simulink model "KalmanFilterIMU"  (R2020a)
settings: Solver=FixedStepDiscrete  StartTime=0.0  StopTime=Inf  RelTol=1e-3
settings Model: SimulationMode=external  SILPILModeSetting=veronly  ExtModeTrigDuration=2  Creator=vishwasgautam  LastModifiedBy=vishwasgautam
settings OptimizationCC: EnhancedBackFolding=on  PassReuseOutputArgsAs=Individual arguments  ZeroExternalMemoryAtStartup=off  ZeroInternalMemoryAtStartup=off  MaxStackSize=64  OptimizeBlockOrder=speed  DifferentSizesBufferReuse=on  OptimizationCustomize=off  EfficientTunableParamExpr=on
settings DebuggingCC: ParameterTunabilityLossMsg=error
settings HardwareCC: ProdBitPerInt=16  ProdBitPerPointer=16  ProdBitPerSizeT=16  ProdBitPerPtrDiffT=16  ProdLargestAtomicFloat=None  ProdWordSize=8  ProdHWDeviceType=Atmel->AVR  UseEmbeddedCoderFeatures=off  UseSimulinkCoderFeatures=off
settings SFSimCC: MATLABDynamicMemAlloc=off
settings RTWCC: SystemTargetFile=ert.tlc  HardwareBoard=Arduino Uno  TLCOptions=-aInlineSetEventsForThisBaseRateFcn=TLC_FALSE -aSuppressMultiTaskScheduler=TLC_FALSE -aRateBasedStepFcn=1  TemplateMakefile=ert_default_tmf  Toolchain=Arduino AVR
settings CodeAppCC: ForceParamTrailComments=on  IgnoreCustomStorageClasses=off  OperatorAnnotations=on  SimulinkDataObjDesc=on  SFDataObjDesc=on  InsertBlockDesc=on
settings ERTTargetCC: SupportContinuousTime=on  SupportNonInlinedSFcns=on  SupportVariableSizeSignals=on  ExtModeStaticAllocSize=250

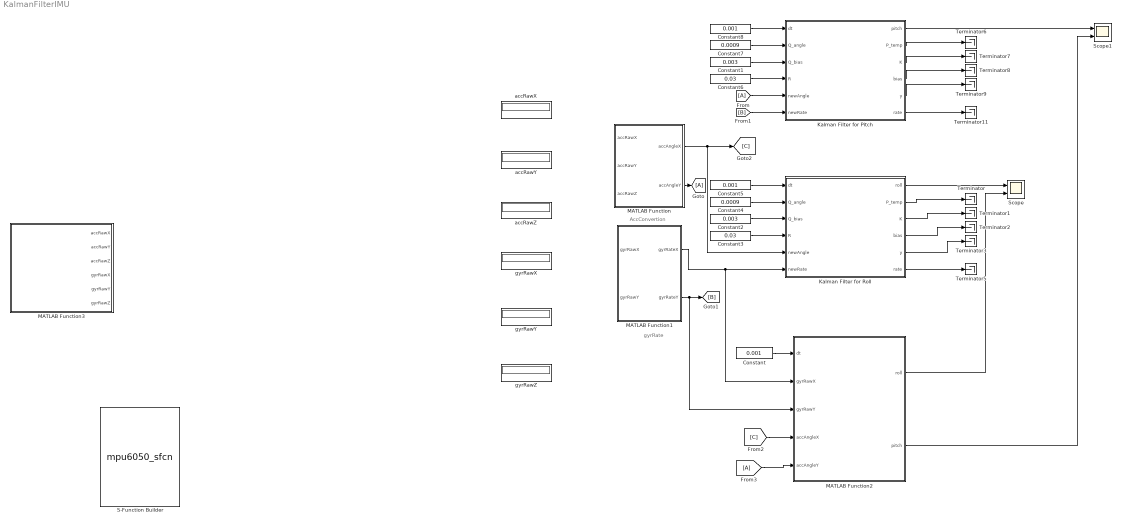
== system KalmanFilterIMU ==
  note: gyrRate
  note: AccConvertion
  Constant : Constant  Value=0.001
  Constant1 : Constant  Value=0.003
  Constant2 : Constant  Value=0.003
  Constant3 : Constant  Value=0.03
  Constant4 : Constant  Value=0.0009
  Constant5 : Constant  Value=0.001
  Constant6 : Constant  Value=0.03
  Constant7 : Constant  Value=0.0009
  Constant8 : Constant  Value=0.001
  Kalman Filter for Pitch : MATLAB Function  TreatAsAtomicUnit=on
  Kalman Filter for Roll : MATLAB Function  TreatAsAtomicUnit=on
  MATLAB Function : MATLAB Function  TreatAsAtomicUnit=on
  MATLAB Function1 : MATLAB Function  TreatAsAtomicUnit=on
  MATLAB Function2 : MATLAB Function  TreatAsAtomicUnit=on
  MATLAB Function3 : MATLAB Function  TreatAsAtomicUnit=on
  S-Function Builder : S-Function  InitFcn=try, set_param(gcb,'FunctionName','mpu6050_sfcn'), end  FunctionName=mpu6050_sfcn  SFunctionModules=mpu6050_sfcn_wrapper  SFunctionDeploymentMode=off  EnableBusSupport=off  mask(S-Function Builder){}
      mask help: Simulink:masks:SFunctionBuilder_MD
      mask init:
      | val = [[.9  0.75 0.75 1 1 .9 .9 1]',[1 1 0.75 0.75 .9 .9 1 .9]'];try , sys = get_param(gcb,'SfunBuilderFcnName');if isempty(sys), sys = get_param(gcb,'FunctionName'); end,catch, sys = get_param(gcb,'FunctionName'); end
      settings: CopyFcn=set_param(gcbh,'LinkStatus','none')  PreSaveFcn=try, set_param(gcb,'FunctionName','mpu6050_sfcn'), end  OpenFcn=sfunctionwizard(gcbh)
      mask Display:
      | plot(val(:,1),val(:,2))
      | disp(sys)
      | port_label('output',1,'accRawX')
      | port_label('output',2,'accRawY')
      | port_label('output',3,'accRawZ')
      | port_label('output',4,'gyrRawX')
      | port_label('output',5,'gyrRawY')
      | port_label('output',6,'gyrRawZ')
  Scope : Scope  NumInputPorts=2
  Scope1 : Scope  NumInputPorts=2
  Terminator{,1..3,5..9,11} (10 alike) : Terminator
  accRawX : Display
      settings: Format=bank
  accRawY : Display
      settings: Format=bank
  accRawZ : Display
      settings: Format=bank
  gyrRawX : Display
      settings: Format=bank
  gyrRawY : Display
      settings: Format=bank
  gyrRawZ : Display
  wires:
  ? -> MATLAB Function/1(accRawX), accRawX/1
  ? -> accRawY/1, MATLAB Function/2(accRawY)
  ? -> MATLAB Function/3(accRawZ), accRawZ/1
  ? -> gyrRawX/1, MATLAB Function1/1(gyrRawX)
  ? -> MATLAB Function1/2(gyrRawY), gyrRawY/1
  ? -> gyrRawZ/1
  MATLAB Function1/1(gyrRateX) -> MATLAB Function2/2(gyrRawX), Kalman Filter for Roll/6(newRate)
  MATLAB Function/1(accAngleX) -> [C], Kalman Filter for Roll/5(newAngle)
  Constant3/1 -> Kalman Filter for Roll/4(R)
  Constant2/1 -> Kalman Filter for Roll/3(Q_bias)
  Constant5/1 -> Kalman Filter for Roll/1(dt)
  Constant4/1 -> Kalman Filter for Roll/2(Q_angle)
  Kalman Filter for Roll/2(P_temp) -> Terminator/1
  Kalman Filter for Roll/3(K) -> Terminator1/1
  Kalman Filter for Roll/4(bias) -> Terminator2/1
  Kalman Filter for Roll/5(y) -> Terminator3/1
  Kalman Filter for Roll/6(rate) -> Terminator5/1
  Kalman Filter for Roll/1(roll) -> Scope/1
  Kalman Filter for Pitch/1(pitch) -> Scope1/1
  Kalman Filter for Pitch/5(y) -> Terminator9/1
  Kalman Filter for Pitch/2(P_temp) -> Terminator6/1
  Kalman Filter for Pitch/4(bias) -> Terminator8/1
  Kalman Filter for Pitch/3(K) -> Terminator7/1
  Kalman Filter for Pitch/6(rate) -> Terminator11/1
  Constant1/1 -> Kalman Filter for Pitch/3(Q_bias)
  Constant8/1 -> Kalman Filter for Pitch/1(dt)
  Constant6/1 -> Kalman Filter for Pitch/4(R)
  Constant7/1 -> Kalman Filter for Pitch/2(Q_angle)
  MATLAB Function/2(accAngleY) -> [A]
  [A] -> Kalman Filter for Pitch/5(newAngle)
  [B] -> Kalman Filter for Pitch/6(newRate)
  MATLAB Function1/2(gyrRateY) -> MATLAB Function2/3(gyrRawY), [B]
  Constant/1 -> MATLAB Function2/1(dt)
  [C] -> MATLAB Function2/4(accAngleX)
  [A] -> MATLAB Function2/5(accAngleY)
  MATLAB Function2/1(roll) -> Scope/2
  MATLAB Function2/2(pitch) -> Scope1/2

== matlab function KalmanFilterIMU/MATLAB Function ==
  data: accRawX input; accAngleX output; accAngleY output; accRawY input; accRawZ input
function [accAngleX, accAngleY] = fcn(accRawX, accRawY, accRawZ)

%Converting the raw accel data from g values to accel about X and Y axis

accAngleX = atan(accRawY/sqrt(power(accRawX,2) + power(accRawZ,2)))*(180/pi);
accAngleY = atan(-1*(accRawX/sqrt(power(accRawY,2) + power(accRawZ,2))))*(180/pi);

end

== matlab function KalmanFilterIMU/MATLAB Function3 ==
  data: accRawX output; accRawY output; accRawZ output; gyrRawX output; gyrRawY output; gyrRawZ output
function [accRawX, accRawY, accRawZ, gyrRawX, gyrRawY, gyrRawZ] = fcn()

a = arduino('/dev/tty.usbmodem143301', 'Uno', 'Libraries', 'I2C');
imu = mpu6050(a);

accelReadings = readAcceleration(imu);

gyroReadings = readAngularVelocity(imu);

accRawX = accelReadings(1);
accRawY = accelReadings(2);
accRawZ = accelReadings(3);

gyrRawX = gyroReadings(1);
gyrRawY = gyroReadings(2);
gyrRawZ = gyroReadings(3);

end

== matlab function KalmanFilterIMU/MATLAB Function1 ==
  data: gyrRawX input; gyrRateX output; gyrRateY output; gyrRawY input
function [gyrRateX, gyrRateY] = fcn(gyrRawX, gyrRawY)

gyrRateX = gyrRawX/131.0;
gyrRateY = gyrRawY/131.0;

end

== matlab function KalmanFilterIMU/Kalman Filter for Roll ==
  data: dt input; roll output; Q_angle input; Q_bias input; R input; newAngle input; newRate input; P_temp output; K output; bias output; y output; rate output
function [roll, P_temp, K, bias, y, rate]  = kalFilterRoll(dt, Q_angle, Q_bias, R, newAngle, newRate)

persistent angle;
persistent P;


%Process Noise Convariance Matrix
Q = [Q_angle 0; 0 Q_bias] * dt;
F = [1  -dt; 0 1];
H = [1 0];
bias = 0.0;

rate = newRate - bias;

if isempty(angle); angle = 0;
    
else angle = angle + (dt * rate);
end 

roll = angle;

if isempty(P); P = [0, 0; 0, 0];
else P = F*P*F' + Q;
end 
P_temp = P;

S = H*P*H' + R;
K = (P_temp * H')/S;
y = newAngle - roll; 
roll = roll + K(1) * y;
bias = roll + K(2) * y;
angle = roll;

I = [1 0; 0 1];
P_temp = (I - K*H)*P_temp;
P = P_temp;

return 


end

== matlab function KalmanFilterIMU/Kalman Filter for Pitch ==
  data: dt input; pitch output; Q_angle input; Q_bias input; R input; newAngle input; newRate input; P_temp output; K output; bias output; y output; rate output
function [pitch, P_temp, K, bias, y, rate]  = kalFilterPitch(dt, Q_angle, Q_bias, R, newAngle, newRate)

persistent angle;
persistent P;


%Process Noise Convariance Matrix
Q = [Q_angle 0; 0 Q_bias] * dt;
F = [1  -dt; 0 1];
H = [1 0];
bias = 0.0;

rate = newRate - bias;

if isempty(angle); angle = 0;
    
else angle = angle + (dt * rate);
end 

pitch = angle;

if isempty(P); P = [0, 0; 0, 0];
else P = F*P*F' + Q;
end 
P_temp = P;

S = H*P*H' + R;
K = (P_temp * H')/S;
y = newAngle - pitch; 
pitch = pitch + K(1) * y;
bias = pitch + K(2) * y;
angle = pitch;

I = [1 0; 0 1];
P_temp = (I - K*H)*P_temp;
P = P_temp;

return 


end

== matlab function KalmanFilterIMU/MATLAB Function2 ==
  data: dt input; roll output; pitch output; gyrRawX input; gyrRawY input; accAngleX input; accAngleY input
function [roll, pitch] = complimentaryF(dt, gyrRawX, gyrRawY, accAngleX, accAngleY)

 gyrAngleX = gyrRawX * dt;
 gyrAngleY = gyrRawY * dt;
 roll = 0.98 * (gyrAngleX) + 0.02 * accAngleX;
 pitch = 0.98 * (gyrAngleY) + 0.02 * accAngleY;
 
end
